simulink model "test_jac_invdyn"  (R2020a)
settings: Solver=ode15s  StartTime=0.0  StopTime=8  RelTol=1e-3
values from neighbouring files (symbols this model uses):
  Kjac = 10*diag([1 1 1 1 1 1])    [JoinScript.m]
  qf = [0 pi/3 pi/12 pi/2 pi/4 0]    [JoinScript.m]    (also in alldata.mat = [1.57079632679 1.0471975512 0.261799387799 1.57079632679 0 1; model_script.m = [pi/6 0 pi/3 pi/4 0 0])
  x0 = [-5.32301496588e-18 0.480120382501 0.16494818601 1.57079632679 -1.04530142769e-16 -2.87979326579]    [alldata.mat]
settings Model: Creator=doble  LastModifiedBy=doble

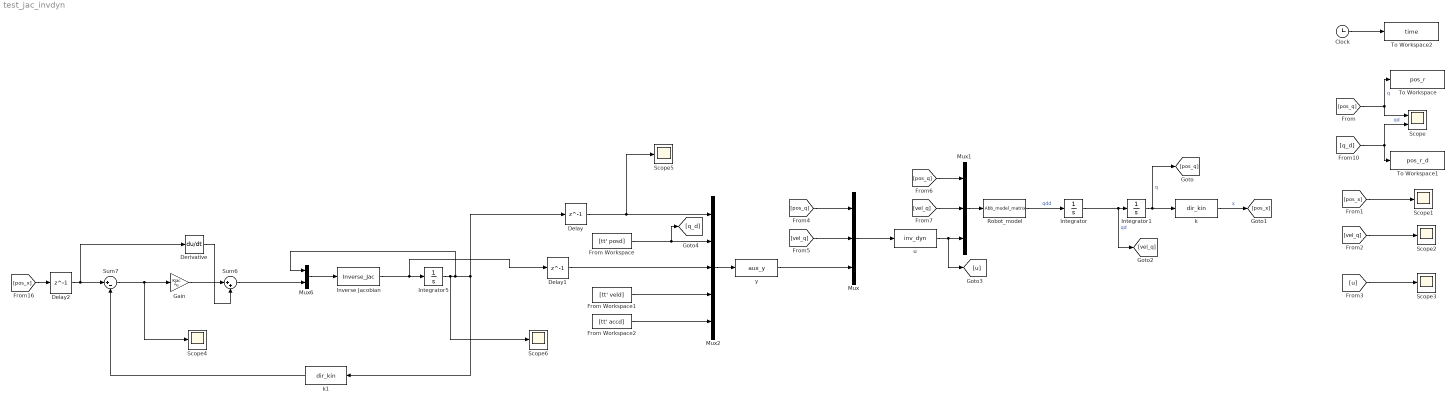
== system test_jac_invdyn ==
  Clock : Clock
  Delay : Delay  DelayLength=1  InitialCondition=x0
  Delay1 : Delay  DelayLength=1
  Delay2 : Delay  DelayLength=1  InitialCondition=x0
  Derivative : Derivative
  From Workspace : FromWorkspace  VariableName=[tt' posd]
  From Workspace1 : FromWorkspace  VariableName=[tt' veld]
  From Workspace2 : FromWorkspace  VariableName=[tt' accd]
  Gain : Gain  Gain=Kjac  Multiplication=Matrix(K*u)
  Integrator : Integrator
  Integrator1 : Integrator  InitialCondition=qf
  Integrator5 : Integrator  InitialCondition=qf
  Inverse Jacobian : MATLABFcn  MATLABFcn=Inverse_Jac  OutputDimensions=6*1
  Mux : Mux  Inputs=[6 6 6]
  Mux1 : Mux  Inputs=[6 6 6]
  Mux2 : Mux  Inputs=[6 6 6 6 6]
  Mux6 : Mux  Inputs=[6 6]
  Robot_model : MATLABFcn  MATLABFcn=Abb_model_matrix  OutputDimensions=6
  Scope : Scope  NumInputPorts=2
  Scope{1..6} (6 alike) : Scope
  Sum6 : Sum  Inputs=|++
  Sum7 : Sum  Inputs=|+-
  To Workspace : ToWorkspace  VariableName=pos_r  SampleTime=-1
  To Workspace1 : ToWorkspace  VariableName=pos_r_d  SampleTime=-1
  To Workspace2 : ToWorkspace  VariableName=time  SampleTime=-1
  k : MATLABFcn  MATLABFcn=dir_kin
  k1 : MATLABFcn  MATLABFcn=dir_kin
  u : MATLABFcn  MATLABFcn=inv_dyn  OutputDimensions=6
  y : MATLABFcn  MATLABFcn=aux_y
  wires:
  [pos_q] -> Mux1/1
  From Workspace/1 -> [q_d], Mux2/2
  u/1 -> Mux1/3, [u]
  Mux2/1 -> y/1
  [pos_q] -> Mux/1
  k/1 -> [pos_x]  "x"
  From Workspace1/1 -> Mux2/4
  Mux1/1 -> Robot_model/1
  [vel_q] -> Mux/2
  Integrator1/1 -> [pos_q], k/1  "q"
  Integrator/1 -> [vel_q], Integrator1/1  "qd"
  Mux/1 -> u/1
  Robot_model/1 -> Integrator/1  "qdd"
  y/1 -> Mux/3
  [u] -> Scope3/1
  [vel_q] -> Mux1/2
  [vel_q] -> Scope2/1
  [q_d] -> To Workspace1/1, Scope/2  "qd"
  Clock/1 -> To Workspace2/1
  [pos_q] -> Scope/1, To Workspace/1  "q"
  From Workspace2/1 -> Mux2/5
  Delay1/1 -> Mux2/3
  Delay/1 -> Mux2/1, Scope5/1
  Integrator5/1 -> Scope6/1, Mux6/1, Delay/1, k1/1
  k1/1 -> Sum7/2
  Sum7/1 -> Scope4/1, Gain/1
  Derivative/1 -> Sum6/2
  Inverse Jacobian/1 -> Delay1/1, Integrator5/1
  Sum6/1 -> Mux6/2
  Mux6/1 -> Inverse Jacobian/1
  Gain/1 -> Sum6/1
  [pos_x] -> Delay2/1
  Delay2/1 -> Derivative/1, Sum7/1
  [pos_x] -> Scope1/1
